simulink model "PassengerCar"  (R2019b)
settings: Solver=ode1  StartTime=0  StopTime=25  FixedStep=1.0000000000000000e-003  RelTol=1e-3
InitFcn:
  | sampleTime = str2double(get_param(bdroot, 'FixedStep'));
undefined symbols (not defined in the file or in its folder): AccPedalPos, BrakePedalPos, BrakeSwitch, DiscIntNeverNeededParam, DYNA4, EngSpd, IgnitionSwitch, InitialGear, InitialSpeed, IntendedEngTrq, LeftIndicator, MainBrakePress, MaxGear, MDL, MinGear, RefAcc, RefLane, RefLatPos, RefPath, RefPathCurv, RefSpd, RefSpdPreview, RefSpdRetrospect, RightIndicator, SteeringWheelAng, SteeringWheelTrq, UserDefinedRefValue, vm_const
libraries: UtilitiesLibrary x31, simulink x18, WheelSystemModules x13, LongitudinalControllerModules x13, LateralControllerModules x7, AnimationBusselectorModules x5, EnvironmentModules x5, BasicEngineControlModules x5, MiscellaneousControlModules x5, Animation3Modules x4, AuxiliariesModules x4, TireModules x4
(part 35 of 39)

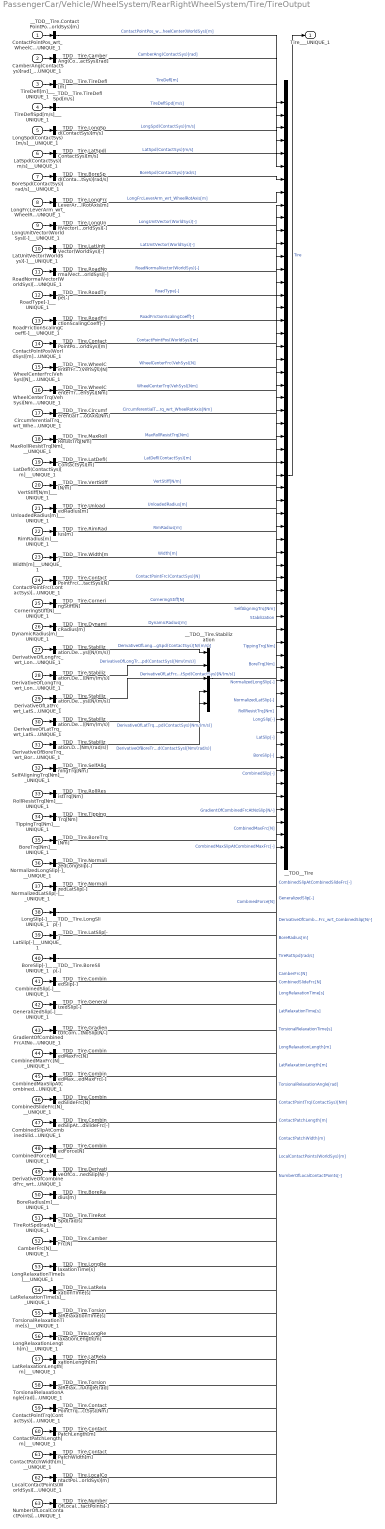
== system PassengerCar/Vehicle/WheelSystem/RearRightWheelSystem/Tire/TireOutput ==
  ContactPointPos_wrt_WheelCenter(WorldSys)[m]___UNIQUE_1 : Inport  Description=|  PortDimensions=[3]
      | <name>ContactPointPos_wrt_WheelCenter(WorldSys)[m]</name>
      | <comment></comment>
  CamberAng(ContactSys)[rad]___UNIQUE_1 : Inport  Description=|  Port=2  PortDimensions=[1]
      | <name>CamberAng(ContactSys)[rad]</name>
      | <comment></comment>
  TireDefl[m]___UNIQUE_1 : Inport  Description=|  Port=3  PortDimensions=[1]
      | <name>TireDefl[m]</name>
      | <comment></comment>
  TireDeflSpd[m/s]___UNIQUE_1 : Inport  Description=|  Port=4  PortDimensions=[1]
      | <name>TireDeflSpd[m/s]</name>
      | <comment></comment>
  LongSpd(ContactSys)[m/s]___UNIQUE_1 : Inport  Description=|  Port=5  PortDimensions=[1]
      | <name>LongSpd(ContactSys)[m/s]</name>
      | <comment></comment>
  LatSpd(ContactSys)[m/s]___UNIQUE_1 : Inport  Description=|  Port=6  PortDimensions=[1]
      | <name>LatSpd(ContactSys)[m/s]</name>
      | <comment></comment>
  BoreSpd(ContactSys)[rad/s]___UNIQUE_1 : Inport  Description=|  Port=7  PortDimensions=[1]
      | <name>BoreSpd(ContactSys)[rad/s]</name>
      | <comment></comment>
  LongFrcLeverArm_wrt_WheelRotAxis[m]___UNIQUE_1 : Inport  Description=|  Port=8  PortDimensions=[1]
      | <name>LongFrcLeverArm_wrt_WheelRotAxis[m]</name>
      | <comment></comment>
  LongUnitVector(WorldSys)[-]___UNIQUE_1 : Inport  Description=|  Port=9  PortDimensions=[3]
      | <name>LongUnitVector(WorldSys)[-]</name>
      | <comment></comment>
  LatUnitVector(WorldSys)[-]___UNIQUE_1 : Inport  Description=|  Port=10  PortDimensions=[3]
      | <name>LatUnitVector(WorldSys)[-]</name>
      | <comment></comment>
  RoadNormalVector(WorldSys)[-]___UNIQUE_1 : Inport  Description=|  Port=11  PortDimensions=[3]
      | <name>RoadNormalVector(WorldSys)[-]</name>
      | <comment></comment>
  RoadType[-]___UNIQUE_1 : Inport  Description=|  Port=12  PortDimensions=[1]
      | <name>RoadType[-]</name>
      | <comment></comment>
  RoadFrictionScalingCoeff[-]___UNIQUE_1 : Inport  Description=|  Port=13  PortDimensions=[1]
      | <name>RoadFrictionScalingCoeff[-]</name>
      | <comment></comment>
  ContactPointPos(WorldSys)[m]___UNIQUE_1 : Inport  Description=|  Port=14  PortDimensions=[3]
      | <name>ContactPointPos(WorldSys)[m]</name>
      | <comment></comment>
  WheelCenterFrc(VehSys)[N]___UNIQUE_1 : Inport  Description=|  Port=15  PortDimensions=[3]
      | <name>WheelCenterFrc(VehSys)[N]</name>
      | <comment></comment>
  WheelCenterTrq(VehSys)[Nm]___UNIQUE_1 : Inport  Description=|  Port=16  PortDimensions=[3]
      | <name>WheelCenterTrq(VehSys)[Nm]</name>
      | <comment></comment>
  CircumferentialTrq_wrt_WheelRotAxis[Nm]___UNIQUE_1 : Inport  Description=|  Port=17  PortDimensions=[1]
      | <name>CircumferentialTrq_wrt_WheelRotAxis[Nm]</name>
      | <comment></comment>
  MaxRollResistTrq[Nm]___UNIQUE_1 : Inport  Description=|  Port=18  PortDimensions=[1]
      | <name>MaxRollResistTrq[Nm]</name>
      | <comment></comment>
  LatDefl(ContactSys)[m]___UNIQUE_1 : Inport  Description=|  Port=19  PortDimensions=[1]
      | <name>LatDefl(ContactSys)[m]</name>
      | <comment></comment>
  VertStiff[N/m]___UNIQUE_1 : Inport  Description=|  Port=20  PortDimensions=[1]
      | <name>VertStiff[N/m]</name>
      | <comment></comment>
  UnloadedRadius[m]___UNIQUE_1 : Inport  Description=|  Port=21  PortDimensions=[1]
      | <name>UnloadedRadius[m]</name>
      | <comment></comment>
  RimRadius[m]___UNIQUE_1 : Inport  Description=|  Port=22  PortDimensions=[1]
      | <name>RimRadius[m]</name>
      | <comment></comment>
  Width[m]___UNIQUE_1 : Inport  Description=|  Port=23  PortDimensions=[1]
      | <name>Width[m]</name>
      | <comment></comment>
  ContactPointFrc(ContactSys)[N]___UNIQUE_1 : Inport  Description=|  Port=24  PortDimensions=[3]
      | <name>ContactPointFrc(ContactSys)[N]</name>
      | <comment></comment>
  CorneringStiff[N]___UNIQUE_1 : Inport  Description=|  Port=25  PortDimensions=[1]
      | <name>CorneringStiff[N]</name>
      | <comment></comment>
  DynamicRadius[m]___UNIQUE_1 : Inport  Description=|  Port=26  PortDimensions=[1]
      | <name>DynamicRadius[m]</name>
      | <comment></comment>
  DerivativeOfLongFrc_wrt_LongSpd(ContactSys)[N/(m/s)]___UNIQUE_1 : Inport  Description=|  Port=27  PortDimensions=[1]
      | <name>Stabilization.DerivativeOfLongFrc_wrt_LongSpd(ContactSys)[N/(m/s)]</name>
      | <comment></comment>
  DerivativeOfLongTrq_wrt_LongSpd(ContactSys)[Nm/(m/s)]___UNIQUE_1 : Inport  Description=|  Port=28  PortDimensions=[1]
      | <name>Stabilization.DerivativeOfLongTrq_wrt_LongSpd(ContactSys)[Nm/(m/s)]</name>
      | <comment></comment>
  DerivativeOfLatFrc_wrt_LatSpd(ContactSys)[N/(m/s)]___UNIQUE_1 : Inport  Description=|  Port=29  PortDimensions=[1]
      | <name>Stabilization.DerivativeOfLatFrc_wrt_LatSpd(ContactSys)[N/(m/s)]</name>
      | <comment></comment>
  DerivativeOfLatTrq_wrt_LatSpd(ContactSys)[Nm/(m/s)]___UNIQUE_1 : Inport  Description=|  Port=30  PortDimensions=[1]
      | <name>Stabilization.DerivativeOfLatTrq_wrt_LatSpd(ContactSys)[Nm/(m/s)]</name>
      | <comment></comment>
  DerivativeOfBoreTrq_wrt_BoreSpd(ContactSys)[Nm/(rad/s)]___UNIQUE_1 : Inport  Description=|  Port=31  PortDimensions=[1]
      | <name>Stabilization.DerivativeOfBoreTrq_wrt_BoreSpd(ContactSys)[Nm/(rad/s)]</name>
      | <comment></comment>
  SelfAligningTrq[Nm]___UNIQUE_1 : Inport  Description=|  Port=32  PortDimensions=[1]
      | <name>SelfAligningTrq[Nm]</name>
      | <comment></comment>
  RollResistTrq[Nm]___UNIQUE_1 : Inport  Description=|  Port=33  PortDimensions=[1]
      | <name>RollResistTrq[Nm]</name>
      | <comment></comment>
  TippingTrq[Nm]___UNIQUE_1 : Inport  Description=|  Port=34  PortDimensions=[1]
      | <name>TippingTrq[Nm]</name>
      | <comment></comment>
  BoreTrq[Nm]___UNIQUE_1 : Inport  Description=|  Port=35  PortDimensions=[1]
      | <name>BoreTrq[Nm]</name>
      | <comment></comment>
  NormalizedLongSlip[-]___UNIQUE_1 : Inport  Description=|  Port=36  PortDimensions=[1]
      | <name>NormalizedLongSlip[-]</name>
      | <comment></comment>
  NormalizedLatSlip[-]___UNIQUE_1 : Inport  Description=|  Port=37  PortDimensions=[1]
      | <name>NormalizedLatSlip[-]</name>
      | <comment></comment>
  LongSlip[-]___UNIQUE_1 : Inport  Description=|  Port=38  PortDimensions=[1]
      | <name>LongSlip[-]</name>
      | <comment></comment>
  LatSlip[-]___UNIQUE_1 : Inport  Description=|  Port=39  PortDimensions=[1]
      | <name>LatSlip[-]</name>
      | <comment></comment>
  BoreSlip[-]___UNIQUE_1 : Inport  Description=|  Port=40  PortDimensions=[1]
      | <name>BoreSlip[-]</name>
      | <comment></comment>
  CombinedSlip[-]___UNIQUE_1 : Inport  Description=|  Port=41  PortDimensions=[1]
      | <name>CombinedSlip[-]</name>
      | <comment></comment>
  GeneralizedSlip[-]___UNIQUE_1 : Inport  Description=|  Port=42  PortDimensions=[1]
      | <name>GeneralizedSlip[-]</name>
      | <comment></comment>
  GradientOfCombinedFrcAtNoSlip[N/-]___UNIQUE_1 : Inport  Description=|  Port=43  PortDimensions=[1]
      | <name>GradientOfCombinedFrcAtNoSlip[N/-]</name>
      | <comment></comment>
  CombinedMaxFrc[N]___UNIQUE_1 : Inport  Description=|  Port=44  PortDimensions=[1]
      | <name>CombinedMaxFrc[N]</name>
      | <comment></comment>
  CombinedMaxSlipAtCombinedMaxFrc[-]___UNIQUE_1 : Inport  Description=|  Port=45  PortDimensions=[1]
      | <name>CombinedMaxSlipAtCombinedMaxFrc[-]</name>
      | <comment></comment>
  CombinedSlideFrc[N]___UNIQUE_1 : Inport  Description=|  Port=46  PortDimensions=[1]
      | <name>CombinedSlideFrc[N]</name>
      | <comment></comment>
  CombinedSlipAtCombinedSlideFrc[-]___UNIQUE_1 : Inport  Description=|  Port=47  PortDimensions=[1]
      | <name>CombinedSlipAtCombinedSlideFrc[-]</name>
      | <comment></comment>
  CombinedForce[N]___UNIQUE_1 : Inport  Description=|  Port=48  PortDimensions=[1]
      | <name>CombinedForce[N]</name>
      | <comment></comment>
  DerivativeOfCombinedFrc_wrt_CombinedSlip[N/-]___UNIQUE_1 : Inport  Description=|  Port=49  PortDimensions=[1]
      | <name>DerivativeOfCombinedFrc_wrt_CombinedSlip[N/-]</name>
      | <comment></comment>
  BoreRadius[m]___UNIQUE_1 : Inport  Description=|  Port=50  PortDimensions=[1]
      | <name>BoreRadius[m]</name>
      | <comment></comment>
  TireRotSpd[rad/s]___UNIQUE_1 : Inport  Description=|  Port=51  PortDimensions=[1]
      | <name>TireRotSpd[rad/s]</name>
      | <comment></comment>
  CamberFrc[N]___UNIQUE_1 : Inport  Description=|  Port=52  PortDimensions=[1]
      | <name>CamberFrc[N]</name>
      | <comment></comment>
  LongRelaxationTime[s]___UNIQUE_1 : Inport  Description=|  Port=53  PortDimensions=[1]
      | <name>LongRelaxationTime[s]</name>
      | <comment></comment>
  LatRelaxationTime[s]___UNIQUE_1 : Inport  Description=|  Port=54  PortDimensions=[1]
      | <name>LatRelaxationTime[s]</name>
      | <comment></comment>
  TorsionalRelaxationTime[s]___UNIQUE_1 : Inport  Description=|  Port=55  PortDimensions=[1]
      | <name>TorsionalRelaxationTime[s]</name>
      | <comment></comment>
  LongRelaxationLength[m]___UNIQUE_1 : Inport  Description=|  Port=56  PortDimensions=[1]
      | <name>LongRelaxationLength[m]</name>
      | <comment></comment>
  LatRelaxationLength[m]___UNIQUE_1 : Inport  Description=|  Port=57  PortDimensions=[1]
      | <name>LatRelaxationLength[m]</name>
      | <comment></comment>
  TorsionalRelaxationAngle[rad]___UNIQUE_1 : Inport  Description=|  Port=58  PortDimensions=[1]
      | <name>TorsionalRelaxationAngle[rad]</name>
      | <comment></comment>
  ContactPointTrq(ContactSys)[Nm]___UNIQUE_1 : Inport  Description=|  Port=59  PortDimensions=[3]
      | <name>ContactPointTrq(ContactSys)[Nm]</name>
      | <comment></comment>
  ContactPatchLength[m]___UNIQUE_1 : Inport  Description=|  Port=60  PortDimensions=[1]
      | <name>ContactPatchLength[m]</name>
      | <comment></comment>
  ContactPatchWidth[m]___UNIQUE_1 : Inport  Description=|  Port=61  PortDimensions=[1]
      | <name>ContactPatchWidth[m]</name>
      | <comment></comment>
  LocalContactPoints(WorldSys)[m]___UNIQUE_1 : Inport  Description=|  Port=62  PortDimensions=[12]
      | <name>LocalContactPoints(WorldSys)[m]</name>
      | <comment></comment>
  NumberOfLocalContactPoints[-]___UNIQUE_1 : Inport  Description=|  Port=63  PortDimensions=[1]
      | <name>NumberOfLocalContactPoints[-]</name>
      | <comment></comment>
  __TDD__Tire.BoreRadius[m] : Demux  Outputs=[1]
  __TDD__Tire.BoreSlip[-] : Demux  Outputs=[1]
  __TDD__Tire.BoreSpd(ContactSys)[rad/s] : Demux  Outputs=[1]
  __TDD__Tire.BoreTrq[Nm] : Demux  Outputs=[1]
  __TDD__Tire.CamberAng(ContactSys)[rad] : Demux  Outputs=[1]
  __TDD__Tire.CamberFrc[N] : Demux  Outputs=[1]
  __TDD__Tire.CircumferentialTrq_wrt_WheelRotAxis[Nm] : Demux  Outputs=[1]
  __TDD__Tire.CombinedForce[N] : Demux  Outputs=[1]
  __TDD__Tire.CombinedMaxFrc[N] : Demux  Outputs=[1]
  __TDD__Tire.CombinedMaxSlipAtCombinedMaxFrc[-] : Demux  Outputs=[1]
  __TDD__Tire.CombinedSlideFrc[N] : Demux  Outputs=[1]
  __TDD__Tire.CombinedSlipAtCombinedSlideFrc[-] : Demux  Outputs=[1]
  __TDD__Tire.CombinedSlip[-] : Demux  Outputs=[1]
  __TDD__Tire.ContactPatchLength[m] : Demux  Outputs=[1]
  __TDD__Tire.ContactPatchWidth[m] : Demux  Outputs=[1]
  __TDD__Tire.ContactPointFrc(ContactSys)[N] : Demux  Outputs=[3]
  __TDD__Tire.ContactPointPos(WorldSys)[m] : Demux  Outputs=[3]
  __TDD__Tire.ContactPointPos_wrt_WheelCenter(WorldSys)[m] : Demux  Outputs=[3]
  __TDD__Tire.ContactPointTrq(ContactSys)[Nm] : Demux  Outputs=[3]
  __TDD__Tire.CorneringStiff[N] : Demux  Outputs=[1]
  __TDD__Tire.DerivativeOfCombinedFrc_wrt_CombinedSlip[N/-] : Demux  Outputs=[1]
  __TDD__Tire.DynamicRadius[m] : Demux  Outputs=[1]
  __TDD__Tire.GeneralizedSlip[-] : Demux  Outputs=[1]
  __TDD__Tire.GradientOfCombinedFrcAtNoSlip[N/-] : Demux  Outputs=[1]
  __TDD__Tire.LatDefl(ContactSys)[m] : Demux  Outputs=[1]
  __TDD__Tire.LatRelaxationLength[m] : Demux  Outputs=[1]
  __TDD__Tire.LatRelaxationTime[s] : Demux  Outputs=[1]
  __TDD__Tire.LatSlip[-] : Demux  Outputs=[1]
  __TDD__Tire.LatSpd(ContactSys)[m/s] : Demux  Outputs=[1]
  __TDD__Tire.LatUnitVector(WorldSys)[-] : Demux  Outputs=[3]
  __TDD__Tire.LocalContactPoints(WorldSys)[m] : Demux  Outputs=[12]
  __TDD__Tire.LongFrcLeverArm_wrt_WheelRotAxis[m] : Demux  Outputs=[1]
  __TDD__Tire.LongRelaxationLength[m] : Demux  Outputs=[1]
  __TDD__Tire.LongRelaxationTime[s] : Demux  Outputs=[1]
  __TDD__Tire.LongSlip[-] : Demux  Outputs=[1]
  __TDD__Tire.LongSpd(ContactSys)[m/s] : Demux  Outputs=[1]
  __TDD__Tire.LongUnitVector(WorldSys)[-] : Demux  Outputs=[3]
  __TDD__Tire.MaxRollResistTrq[Nm] : Demux  Outputs=[1]
  __TDD__Tire.NormalizedLatSlip[-] : Demux  Outputs=[1]
  __TDD__Tire.NormalizedLongSlip[-] : Demux  Outputs=[1]
  __TDD__Tire.NumberOfLocalContactPoints[-] : Demux  Outputs=[1]
  __TDD__Tire.RimRadius[m] : Demux  Outputs=[1]
  __TDD__Tire.RoadFrictionScalingCoeff[-] : Demux  Outputs=[1]
  __TDD__Tire.RoadNormalVector(WorldSys)[-] : Demux  Outputs=[3]
  __TDD__Tire.RoadType[-] : Demux  Outputs=[1]
  __TDD__Tire.RollResistTrq[Nm] : Demux  Outputs=[1]
  __TDD__Tire.SelfAligningTrq[Nm] : Demux  Outputs=[1]
  __TDD__Tire.Stabilization.DerivativeOfBoreTrq_wrt_BoreSpd(ContactSys)[Nm/(rad/s)] : Demux  Outputs=[1]
  __TDD__Tire.Stabilization.DerivativeOfLatFrc_wrt_LatSpd(ContactSys)[N/(m/s)] : Demux  Outputs=[1]
  __TDD__Tire.Stabilization.DerivativeOfLatTrq_wrt_LatSpd(ContactSys)[Nm/(m/s)] : Demux  Outputs=[1]
  __TDD__Tire.Stabilization.DerivativeOfLongFrc_wrt_LongSpd(ContactSys)[N/(m/s)] : Demux  Outputs=[1]
  __TDD__Tire.Stabilization.DerivativeOfLongTrq_wrt_LongSpd(ContactSys)[Nm/(m/s)] : Demux  Outputs=[1]
  __TDD__Tire.TippingTrq[Nm] : Demux  Outputs=[1]
  __TDD__Tire.TireDeflSpd[m/s] : Demux  Outputs=[1]
  __TDD__Tire.TireDefl[m] : Demux  Outputs=[1]
  __TDD__Tire.TireRotSpd[rad/s] : Demux  Outputs=[1]
  __TDD__Tire.TorsionalRelaxationAngle[rad] : Demux  Outputs=[1]
  __TDD__Tire.TorsionalRelaxationTime[s] : Demux  Outputs=[1]
  __TDD__Tire.UnloadedRadius[m] : Demux  Outputs=[1]
  __TDD__Tire.VertStiff[N/m] : Demux  Outputs=[1]
  __TDD__Tire.WheelCenterFrc(VehSys)[N] : Demux  Outputs=[3]
  __TDD__Tire.WheelCenterTrq(VehSys)[Nm] : Demux  Outputs=[3]
  __TDD__Tire.Width[m] : Demux  Outputs=[1]
  __TDO__Tire : BusCreator  Inputs=59
  __TDO__Tire.Stabilization : BusCreator  Inputs=5
  Tire___UNIQUE_1 : Outport  Description=|  PortDimensions=[92]  VectorParamsAs1DForOutWhenUnconnected=off
      | <name>ContactPointPos_wrt_WheelCenter(WorldSys)[m]</name>
      | <comment></comment>
  wires:
  ContactPointPos_wrt_WheelCenter(WorldSys)[m]___UNIQUE_1/1 -> __TDD__Tire.ContactPointPos_wrt_WheelCenter(WorldSys)[m]/1
  __TDD__Tire.ContactPointPos_wrt_WheelCenter(WorldSys)[m]/1 -> __TDO__Tire/1  "ContactPointPos_wrt_WheelCenter(WorldSys)[m]"
  CamberAng(ContactSys)[rad]___UNIQUE_1/1 -> __TDD__Tire.CamberAng(ContactSys)[rad]/1
  __TDD__Tire.CamberAng(ContactSys)[rad]/1 -> __TDO__Tire/2  "CamberAng(ContactSys)[rad]"
  TireDefl[m]___UNIQUE_1/1 -> __TDD__Tire.TireDefl[m]/1
  __TDD__Tire.TireDefl[m]/1 -> __TDO__Tire/3  "TireDefl[m]"
  TireDeflSpd[m/s]___UNIQUE_1/1 -> __TDD__Tire.TireDeflSpd[m/s]/1
  __TDD__Tire.TireDeflSpd[m/s]/1 -> __TDO__Tire/4  "TireDeflSpd[m/s]"
  LongSpd(ContactSys)[m/s]___UNIQUE_1/1 -> __TDD__Tire.LongSpd(ContactSys)[m/s]/1
  __TDD__Tire.LongSpd(ContactSys)[m/s]/1 -> __TDO__Tire/5  "LongSpd(ContactSys)[m/s]"
  LatSpd(ContactSys)[m/s]___UNIQUE_1/1 -> __TDD__Tire.LatSpd(ContactSys)[m/s]/1
  __TDD__Tire.LatSpd(ContactSys)[m/s]/1 -> __TDO__Tire/6  "LatSpd(ContactSys)[m/s]"
  BoreSpd(ContactSys)[rad/s]___UNIQUE_1/1 -> __TDD__Tire.BoreSpd(ContactSys)[rad/s]/1
  __TDD__Tire.BoreSpd(ContactSys)[rad/s]/1 -> __TDO__Tire/7  "BoreSpd(ContactSys)[rad/s]"
  LongFrcLeverArm_wrt_WheelRotAxis[m]___UNIQUE_1/1 -> __TDD__Tire.LongFrcLeverArm_wrt_WheelRotAxis[m]/1
  __TDD__Tire.LongFrcLeverArm_wrt_WheelRotAxis[m]/1 -> __TDO__Tire/8  "LongFrcLeverArm_wrt_WheelRotAxis[m]"
  LongUnitVector(WorldSys)[-]___UNIQUE_1/1 -> __TDD__Tire.LongUnitVector(WorldSys)[-]/1
  __TDD__Tire.LongUnitVector(WorldSys)[-]/1 -> __TDO__Tire/9  "LongUnitVector(WorldSys)[-]"
  LatUnitVector(WorldSys)[-]___UNIQUE_1/1 -> __TDD__Tire.LatUnitVector(WorldSys)[-]/1
  __TDD__Tire.LatUnitVector(WorldSys)[-]/1 -> __TDO__Tire/10  "LatUnitVector(WorldSys)[-]"
  RoadNormalVector(WorldSys)[-]___UNIQUE_1/1 -> __TDD__Tire.RoadNormalVector(WorldSys)[-]/1
  __TDD__Tire.RoadNormalVector(WorldSys)[-]/1 -> __TDO__Tire/11  "RoadNormalVector(WorldSys)[-]"
  RoadType[-]___UNIQUE_1/1 -> __TDD__Tire.RoadType[-]/1
  __TDD__Tire.RoadType[-]/1 -> __TDO__Tire/12  "RoadType[-]"
  RoadFrictionScalingCoeff[-]___UNIQUE_1/1 -> __TDD__Tire.RoadFrictionScalingCoeff[-]/1
  __TDD__Tire.RoadFrictionScalingCoeff[-]/1 -> __TDO__Tire/13  "RoadFrictionScalingCoeff[-]"
  ContactPointPos(WorldSys)[m]___UNIQUE_1/1 -> __TDD__Tire.ContactPointPos(WorldSys)[m]/1
  __TDD__Tire.ContactPointPos(WorldSys)[m]/1 -> __TDO__Tire/14  "ContactPointPos(WorldSys)[m]"
  WheelCenterFrc(VehSys)[N]___UNIQUE_1/1 -> __TDD__Tire.WheelCenterFrc(VehSys)[N]/1
  __TDD__Tire.WheelCenterFrc(VehSys)[N]/1 -> __TDO__Tire/15  "WheelCenterFrc(VehSys)[N]"
  WheelCenterTrq(VehSys)[Nm]___UNIQUE_1/1 -> __TDD__Tire.WheelCenterTrq(VehSys)[Nm]/1
  __TDD__Tire.WheelCenterTrq(VehSys)[Nm]/1 -> __TDO__Tire/16  "WheelCenterTrq(VehSys)[Nm]"
  CircumferentialTrq_wrt_WheelRotAxis[Nm]___UNIQUE_1/1 -> __TDD__Tire.CircumferentialTrq_wrt_WheelRotAxis[Nm]/1
  __TDD__Tire.CircumferentialTrq_wrt_WheelRotAxis[Nm]/1 -> __TDO__Tire/17  "CircumferentialTrq_wrt_WheelRotAxis[Nm]"
  MaxRollResistTrq[Nm]___UNIQUE_1/1 -> __TDD__Tire.MaxRollResistTrq[Nm]/1
  __TDD__Tire.MaxRollResistTrq[Nm]/1 -> __TDO__Tire/18  "MaxRollResistTrq[Nm]"
  LatDefl(ContactSys)[m]___UNIQUE_1/1 -> __TDD__Tire.LatDefl(ContactSys)[m]/1
  __TDD__Tire.LatDefl(ContactSys)[m]/1 -> __TDO__Tire/19  "LatDefl(ContactSys)[m]"
  VertStiff[N/m]___UNIQUE_1/1 -> __TDD__Tire.VertStiff[N/m]/1
  __TDD__Tire.VertStiff[N/m]/1 -> __TDO__Tire/20  "VertStiff[N/m]"
  UnloadedRadius[m]___UNIQUE_1/1 -> __TDD__Tire.UnloadedRadius[m]/1
  __TDD__Tire.UnloadedRadius[m]/1 -> __TDO__Tire/21  "UnloadedRadius[m]"
  RimRadius[m]___UNIQUE_1/1 -> __TDD__Tire.RimRadius[m]/1
  __TDD__Tire.RimRadius[m]/1 -> __TDO__Tire/22  "RimRadius[m]"
  Width[m]___UNIQUE_1/1 -> __TDD__Tire.Width[m]/1
  __TDD__Tire.Width[m]/1 -> __TDO__Tire/23  "Width[m]"
  ContactPointFrc(ContactSys)[N]___UNIQUE_1/1 -> __TDD__Tire.ContactPointFrc(ContactSys)[N]/1
  __TDD__Tire.ContactPointFrc(ContactSys)[N]/1 -> __TDO__Tire/24  "ContactPointFrc(ContactSys)[N]"
  CorneringStiff[N]___UNIQUE_1/1 -> __TDD__Tire.CorneringStiff[N]/1
  __TDD__Tire.CorneringStiff[N]/1 -> __TDO__Tire/25  "CorneringStiff[N]"
  DynamicRadius[m]___UNIQUE_1/1 -> __TDD__Tire.DynamicRadius[m]/1
  __TDD__Tire.DynamicRadius[m]/1 -> __TDO__Tire/26  "DynamicRadius[m]"
  DerivativeOfLongFrc_wrt_LongSpd(ContactSys)[N/(m/s)]___UNIQUE_1/1 -> __TDD__Tire.Stabilization.DerivativeOfLongFrc_wrt_LongSpd(ContactSys)[N/(m/s)]/1
  __TDD__Tire.Stabilization.DerivativeOfLongFrc_wrt_LongSpd(ContactSys)[N/(m/s)]/1 -> __TDO__Tire.Stabilization/1  "DerivativeOfLongFrc_wrt_LongSpd(ContactSys)[N/(m/s)]"
  __TDO__Tire.Stabilization/1 -> __TDO__Tire/27  "Stabilization"
  DerivativeOfLongTrq_wrt_LongSpd(ContactSys)[Nm/(m/s)]___UNIQUE_1/1 -> __TDD__Tire.Stabilization.DerivativeOfLongTrq_wrt_LongSpd(ContactSys)[Nm/(m/s)]/1
  __TDD__Tire.Stabilization.DerivativeOfLongTrq_wrt_LongSpd(ContactSys)[Nm/(m/s)]/1 -> __TDO__Tire.Stabilization/2  "DerivativeOfLongTrq_wrt_LongSpd(ContactSys)[Nm/(m/s)]"
  DerivativeOfLatFrc_wrt_LatSpd(ContactSys)[N/(m/s)]___UNIQUE_1/1 -> __TDD__Tire.Stabilization.DerivativeOfLatFrc_wrt_LatSpd(ContactSys)[N/(m/s)]/1
  __TDD__Tire.Stabilization.DerivativeOfLatFrc_wrt_LatSpd(ContactSys)[N/(m/s)]/1 -> __TDO__Tire.Stabilization/3  "DerivativeOfLatFrc_wrt_LatSpd(ContactSys)[N/(m/s)]"
  DerivativeOfLatTrq_wrt_LatSpd(ContactSys)[Nm/(m/s)]___UNIQUE_1/1 -> __TDD__Tire.Stabilization.DerivativeOfLatTrq_wrt_LatSpd(ContactSys)[Nm/(m/s)]/1
  __TDD__Tire.Stabilization.DerivativeOfLatTrq_wrt_LatSpd(ContactSys)[Nm/(m/s)]/1 -> __TDO__Tire.Stabilization/4  "DerivativeOfLatTrq_wrt_LatSpd(ContactSys)[Nm/(m/s)]"
  DerivativeOfBoreTrq_wrt_BoreSpd(ContactSys)[Nm/(rad/s)]___UNIQUE_1/1 -> __TDD__Tire.Stabilization.DerivativeOfBoreTrq_wrt_BoreSpd(ContactSys)[Nm/(rad/s)]/1
  __TDD__Tire.Stabilization.DerivativeOfBoreTrq_wrt_BoreSpd(ContactSys)[Nm/(rad/s)]/1 -> __TDO__Tire.Stabilization/5  "DerivativeOfBoreTrq_wrt_BoreSpd(ContactSys)[Nm/(rad/s)]"
  SelfAligningTrq[Nm]___UNIQUE_1/1 -> __TDD__Tire.SelfAligningTrq[Nm]/1
  __TDD__Tire.SelfAligningTrq[Nm]/1 -> __TDO__Tire/28  "SelfAligningTrq[Nm]"
  RollResistTrq[Nm]___UNIQUE_1/1 -> __TDD__Tire.RollResistTrq[Nm]/1
  __TDD__Tire.RollResistTrq[Nm]/1 -> __TDO__Tire/29  "RollResistTrq[Nm]"
  TippingTrq[Nm]___UNIQUE_1/1 -> __TDD__Tire.TippingTrq[Nm]/1
  __TDD__Tire.TippingTrq[Nm]/1 -> __TDO__Tire/30  "TippingTrq[Nm]"
  BoreTrq[Nm]___UNIQUE_1/1 -> __TDD__Tire.BoreTrq[Nm]/1
  __TDD__Tire.BoreTrq[Nm]/1 -> __TDO__Tire/31  "BoreTrq[Nm]"
  NormalizedLongSlip[-]___UNIQUE_1/1 -> __TDD__Tire.NormalizedLongSlip[-]/1
  __TDD__Tire.NormalizedLongSlip[-]/1 -> __TDO__Tire/32  "NormalizedLongSlip[-]"
  NormalizedLatSlip[-]___UNIQUE_1/1 -> __TDD__Tire.NormalizedLatSlip[-]/1
  __TDD__Tire.NormalizedLatSlip[-]/1 -> __TDO__Tire/33  "NormalizedLatSlip[-]"
  LongSlip[-]___UNIQUE_1/1 -> __TDD__Tire.LongSlip[-]/1
  __TDD__Tire.LongSlip[-]/1 -> __TDO__Tire/34  "LongSlip[-]"
  LatSlip[-]___UNIQUE_1/1 -> __TDD__Tire.LatSlip[-]/1
  __TDD__Tire.LatSlip[-]/1 -> __TDO__Tire/35  "LatSlip[-]"
  BoreSlip[-]___UNIQUE_1/1 -> __TDD__Tire.BoreSlip[-]/1
  __TDD__Tire.BoreSlip[-]/1 -> __TDO__Tire/36  "BoreSlip[-]"
  CombinedSlip[-]___UNIQUE_1/1 -> __TDD__Tire.CombinedSlip[-]/1
  __TDD__Tire.CombinedSlip[-]/1 -> __TDO__Tire/37  "CombinedSlip[-]"
  GeneralizedSlip[-]___UNIQUE_1/1 -> __TDD__Tire.GeneralizedSlip[-]/1
  __TDD__Tire.GeneralizedSlip[-]/1 -> __TDO__Tire/38  "GeneralizedSlip[-]"
  GradientOfCombinedFrcAtNoSlip[N/-]___UNIQUE_1/1 -> __TDD__Tire.GradientOfCombinedFrcAtNoSlip[N/-]/1
  __TDD__Tire.GradientOfCombinedFrcAtNoSlip[N/-]/1 -> __TDO__Tire/39  "GradientOfCombinedFrcAtNoSlip[N/-]"
  CombinedMaxFrc[N]___UNIQUE_1/1 -> __TDD__Tire.CombinedMaxFrc[N]/1
  __TDD__Tire.CombinedMaxFrc[N]/1 -> __TDO__Tire/40  "CombinedMaxFrc[N]"
  CombinedMaxSlipAtCombinedMaxFrc[-]___UNIQUE_1/1 -> __TDD__Tire.CombinedMaxSlipAtCombinedMaxFrc[-]/1
  __TDD__Tire.CombinedMaxSlipAtCombinedMaxFrc[-]/1 -> __TDO__Tire/41  "CombinedMaxSlipAtCombinedMaxFrc[-]"
  CombinedSlideFrc[N]___UNIQUE_1/1 -> __TDD__Tire.CombinedSlideFrc[N]/1
  __TDD__Tire.CombinedSlideFrc[N]/1 -> __TDO__Tire/42  "CombinedSlideFrc[N]"
  CombinedSlipAtCombinedSlideFrc[-]___UNIQUE_1/1 -> __TDD__Tire.CombinedSlipAtCombinedSlideFrc[-]/1
  __TDD__Tire.CombinedSlipAtCombinedSlideFrc[-]/1 -> __TDO__Tire/43  "CombinedSlipAtCombinedSlideFrc[-]"
  CombinedForce[N]___UNIQUE_1/1 -> __TDD__Tire.CombinedForce[N]/1
  __TDD__Tire.CombinedForce[N]/1 -> __TDO__Tire/44  "CombinedForce[N]"
  DerivativeOfCombinedFrc_wrt_CombinedSlip[N/-]___UNIQUE_1/1 -> __TDD__Tire.DerivativeOfCombinedFrc_wrt_CombinedSlip[N/-]/1
  __TDD__Tire.DerivativeOfCombinedFrc_wrt_CombinedSlip[N/-]/1 -> __TDO__Tire/45  "DerivativeOfCombinedFrc_wrt_CombinedSlip[N/-]"
  BoreRadius[m]___UNIQUE_1/1 -> __TDD__Tire.BoreRadius[m]/1
  __TDD__Tire.BoreRadius[m]/1 -> __TDO__Tire/46  "BoreRadius[m]"
  TireRotSpd[rad/s]___UNIQUE_1/1 -> __TDD__Tire.TireRotSpd[rad/s]/1
  __TDD__Tire.TireRotSpd[rad/s]/1 -> __TDO__Tire/47  "TireRotSpd[rad/s]"
  CamberFrc[N]___UNIQUE_1/1 -> __TDD__Tire.CamberFrc[N]/1
  __TDD__Tire.CamberFrc[N]/1 -> __TDO__Tire/48  "CamberFrc[N]"
  LongRelaxationTime[s]___UNIQUE_1/1 -> __TDD__Tire.LongRelaxationTime[s]/1
  __TDD__Tire.LongRelaxationTime[s]/1 -> __TDO__Tire/49  "LongRelaxationTime[s]"
  LatRelaxationTime[s]___UNIQUE_1/1 -> __TDD__Tire.LatRelaxationTime[s]/1
  __TDD__Tire.LatRelaxationTime[s]/1 -> __TDO__Tire/50  "LatRelaxationTime[s]"
  TorsionalRelaxationTime[s]___UNIQUE_1/1 -> __TDD__Tire.TorsionalRelaxationTime[s]/1
  __TDD__Tire.TorsionalRelaxationTime[s]/1 -> __TDO__Tire/51  "TorsionalRelaxationTime[s]"
  LongRelaxationLength[m]___UNIQUE_1/1 -> __TDD__Tire.LongRelaxationLength[m]/1
  __TDD__Tire.LongRelaxationLength[m]/1 -> __TDO__Tire/52  "LongRelaxationLength[m]"
  LatRelaxationLength[m]___UNIQUE_1/1 -> __TDD__Tire.LatRelaxationLength[m]/1
  __TDD__Tire.LatRelaxationLength[m]/1 -> __TDO__Tire/53  "LatRelaxationLength[m]"
  TorsionalRelaxationAngle[rad]___UNIQUE_1/1 -> __TDD__Tire.TorsionalRelaxationAngle[rad]/1
  __TDD__Tire.TorsionalRelaxationAngle[rad]/1 -> __TDO__Tire/54  "TorsionalRelaxationAngle[rad]"
  ContactPointTrq(ContactSys)[Nm]___UNIQUE_1/1 -> __TDD__Tire.ContactPointTrq(ContactSys)[Nm]/1
  __TDD__Tire.ContactPointTrq(ContactSys)[Nm]/1 -> __TDO__Tire/55  "ContactPointTrq(ContactSys)[Nm]"
  ContactPatchLength[m]___UNIQUE_1/1 -> __TDD__Tire.ContactPatchLength[m]/1
  __TDD__Tire.ContactPatchLength[m]/1 -> __TDO__Tire/56  "ContactPatchLength[m]"
  ContactPatchWidth[m]___UNIQUE_1/1 -> __TDD__Tire.ContactPatchWidth[m]/1
  __TDD__Tire.ContactPatchWidth[m]/1 -> __TDO__Tire/57  "ContactPatchWidth[m]"
  LocalContactPoints(WorldSys)[m]___UNIQUE_1/1 -> __TDD__Tire.LocalContactPoints(WorldSys)[m]/1
  __TDD__Tire.LocalContactPoints(WorldSys)[m]/1 -> __TDO__Tire/58  "LocalContactPoints(WorldSys)[m]"
  NumberOfLocalContactPoints[-]___UNIQUE_1/1 -> __TDD__Tire.NumberOfLocalContactPoints[-]/1
  __TDD__Tire.NumberOfLocalContactPoints[-]/1 -> __TDO__Tire/59  "NumberOfLocalContactPoints[-]"
  __TDO__Tire/1 -> Tire___UNIQUE_1/1  "Tire"

== system PassengerCar/VehicleControl/LateralControl/Disabled LateralControl/ControlSystems/Control Systems Parameters ==
  CurvatureControl : Subsystem
      settings: CopyFcn=DYNA4.Internal.ModelCallbacks.Modules.UpdateMaskParameters(gcb);  NameChangeFcn=DYNA4.Internal.ModelCallbacks.Modules.UpdateMaskParameters(gcb);
  PathControl : Subsystem
      settings: CopyFcn=DYNA4.Internal.ModelCallbacks.Modules.UpdateMaskParameters(gcb);  NameChangeFcn=DYNA4.Internal.ModelCallbacks.Modules.UpdateMaskParameters(gcb);

== system PassengerCar/VehicleControl/LateralControl/Disabled LateralControl/ControlSystems/DynaSystemInfo ==

== system PassengerCar/VehicleControl/LateralControl/Disabled LateralControl/ControlSystems/Lateral Controller ==
  User-Defined Control : Subsystem  TreatAsAtomicUnit=on

== system PassengerCar/VehicleControl/LateralControl/Disabled LateralControl/ControlSystems/LateralControlOutput ==
  __SRC__LateralControl.LateralPhase : Constant  Value=0.0  OutDataTypeStr=Inherit: Inherit via back propagation
  __SRC__LateralControl.LeftIndicator : Constant  Value=0.0  OutDataTypeStr=Inherit: Inherit via back propagation
  __SRC__LateralControl.RightIndicator : Constant  Value=0.0  OutDataTypeStr=Inherit: Inherit via back propagation
  __SRC__LateralControl.SteeringWheelAng : Constant  Value=0.0  OutDataTypeStr=Inherit: Inherit via back propagation
  __SRC__LateralControl.SteeringWheelInputSwitch : Constant  Value=0.0  OutDataTypeStr=Inherit: Inherit via back propagation
  __SRC__LateralControl.SteeringWheelTrq : Constant  Value=0.0  OutDataTypeStr=Inherit: Inherit via back propagation
  __SRC__LateralControl.UserDefined1 : Constant  Value=0.0  OutDataTypeStr=Inherit: Inherit via back propagation
  __SRC__LateralControl.UserDefined2 : Constant  Value=0.0  OutDataTypeStr=Inherit: Inherit via back propagation
  __SRC__LateralControl.UserDefinedRefValue : Constant  Value=0.0  OutDataTypeStr=Inherit: Inherit via back propagation
  __TDO__LateralControl : BusCreator  Inputs=9
  LateralControl___UNIQUE_1 : Outport  Description=|  PortDimensions=[9]  VectorParamsAs1DForOutWhenUnconnected=off
      | <name>SteeringWheelAng</name>
      | <comment>Steering wheel angle</comment>
  wires:
  __TDO__LateralControl/1 -> LateralControl___UNIQUE_1/1  "LateralControl"
  __SRC__LateralControl.UserDefined2/1 -> __TDO__LateralControl/9  "UserDefined2[-]"
  __SRC__LateralControl.UserDefined1/1 -> __TDO__LateralControl/8  "UserDefined1[-]"
  __SRC__LateralControl.LateralPhase/1 -> __TDO__LateralControl/7  "LateralPhase[-]"
  __SRC__LateralControl.RightIndicator/1 -> __TDO__LateralControl/6  "RightIndicator[0;1]"
  __SRC__LateralControl.LeftIndicator/1 -> __TDO__LateralControl/5  "LeftIndicator[0;1]"
  __SRC__LateralControl.UserDefinedRefValue/1 -> __TDO__LateralControl/4  "UserDefinedRefValue[-]"
  __SRC__LateralControl.SteeringWheelInputSwitch/1 -> __TDO__LateralControl/3  "SteeringWheelInputSwitch[-]"
  __SRC__LateralControl.SteeringWheelTrq/1 -> __TDO__LateralControl/2  "SteeringWheelTrq[Nm]"
  __SRC__LateralControl.SteeringWheelAng/1 -> __TDO__LateralControl/1  "SteeringWheelAng[rad]"

== system PassengerCar/VehicleControl/LateralControl/Disabled LateralControl/ControlSystemsPreprocessor/Maneuver ==
  DynaModuleInfo : Subsystem  Tag=DynaModuleInfo
      mask init:
      | data = get_param(gcb, 'UserData');
      mask Display: disp(['Type = ', data.type, '\nName = ', char(data.name)]);

== system PassengerCar/VehicleControl/LateralControl/Enabled LateralControl/ControlSystems/Control Systems Parameters ==
  note: TASK_LAT_STEERING_WHEEL_ANG = 1;
      | 	TASK_LAT_STEERING_WHEEL_TORQUE = 2;
      | 	TASK_LAT_PATH_CONTROL = 3;
      | 	TASK_LAT_CURVATURE_CONTROL = 4;
      | 	TASK_LAT_USER_DEFINED = 5;
  TaskIdentifier : Inport
  CtrlSystemsAbscissae : Inport  Port=2
  Bus Selector : BusSelector  OutputSignals=Task
  CurvatureControl : LateralControllerModules/DataContainerCurvatureControl  DATA_NODE=MDL.VehicleControl.LateralControl.ControlSystems.CurvatureControl  PreviewDist=MDL.VehicleControl.LateralControl.ControlSystems.CurvatureControl.PreviewDist  PreviewTime=MDL.VehicleControl.LateralControl.ControlSystems.CurvatureControl.PreviewTime  TargetAimDist=MDL.VehicleControl.LateralControl.ControlSystems.CurvatureControl.TargetAimDist  MaxLeftSteeringRate=MDL.VehicleControl.LateralControl.ControlSystems.CurvatureControl.MaxLeftSteeringRate  MaxRightSteeringRate=MDL.VehicleControl.LateralControl.ControlSystems.CurvatureControl.MaxRightSteeringRate  SteeringAngSmoothTimeConst=MDL.VehicleControl.LateralControl.ControlSystems.CurvatureControl.SteeringAngSmoothTimeConst  LatCtrlGain=MDL.VehicleControl.LateralControl.ControlSystems.CurvatureControl.LatCtrlGain  ControllerDeviationScaling=MDL.VehicleControl.LateralControl.ControlSystems.CurvatureControl.ControllerDeviationScaling  FrontAxleLatStiff=MDL.VehicleControl.LateralControl.ControlSystems.CurvatureControl.FrontAxleLatStiff  RearAxleLatStiff=MDL.VehicleControl.LateralControl.ControlSystems.CurvatureControl.RearAxleLatStiff  RearTiresLatFrcSmoothTimeConst=MDL.VehicleControl.LateralControl.ControlSystems.CurvatureControl.RearTiresLatFrcSmoothTimeConst  RearTiresLatFrcSwitch=MDL.VehicleControl.LateralControl.ControlSystems.CurvatureControl.RearTiresLatFrcSwitch  RearTiresLatFrcScaling=MDL.VehicleControl.LateralControl.ControlSystems.CurvatureControl.RearTiresLatFrcScaling  SmoothingInterval=MDL.VehicleControl.LateralControl.ControlSystems.CurvatureControl.SmoothingInterval  Preview=MDL.VehicleControl.LateralControl.ControlSystems.CurvatureControl.Preview  DrivingSkill=MDL.VehicleControl.LateralControl.ControlSystems.CurvatureControl.DrivingSkill  Smoothness=MDL.VehicleControl.LateralControl.ControlSystems.CurvatureControl.Smoothness
  Merge : Merge
  PathControl : LateralControllerModules/DataContainerPathControl  DATA_NODE=MDL.VehicleControl.LateralControl.ControlSystems.PathControl  PreviewDist=MDL.VehicleControl.LateralControl.ControlSystems.PathControl.PreviewDist  PreviewTime=MDL.VehicleControl.LateralControl.ControlSystems.PathControl.PreviewTime  TargetAimDist=MDL.VehicleControl.LateralControl.ControlSystems.PathControl.TargetAimDist  MaxLeftSteeringRate=MDL.VehicleControl.LateralControl.ControlSystems.PathControl.MaxLeftSteeringRate  MaxRightSteeringRate=MDL.VehicleControl.LateralControl.ControlSystems.PathControl.MaxRightSteeringRate  SteeringAngSmoothTimeConst=MDL.VehicleControl.LateralControl.ControlSystems.PathControl.SteeringAngSmoothTimeConst  LatCtrlGain=MDL.VehicleControl.LateralControl.ControlSystems.PathControl.LatCtrlGain  ControllerDeviationScaling=MDL.VehicleControl.LateralControl.ControlSystems.PathControl.ControllerDeviationScaling  FrontAxleLatStiff=MDL.VehicleControl.LateralControl.ControlSystems.PathControl.FrontAxleLatStiff  RearAxleLatStiff=MDL.VehicleControl.LateralControl.ControlSystems.PathControl.RearAxleLatStiff  RearTiresLatFrcSmoothTimeConst=MDL.VehicleControl.LateralControl.ControlSystems.PathControl.RearTiresLatFrcSmoothTimeConst  RearTiresLatFrcSwitch=MDL.VehicleControl.LateralControl.ControlSystems.PathControl.RearTiresLatFrcSwitch  RearTiresLatFrcScaling=MDL.VehicleControl.LateralControl.ControlSystems.PathControl.RearTiresLatFrcScaling  LaneChangeDurationTime=MDL.VehicleControl.LateralControl.ControlSystems.PathControl.LaneChangeDurationTime  LaneChangeDurationDist=MDL.VehicleControl.LateralControl.ControlSystems.PathControl.LaneChangeDurationDist  SmoothingInterval=MDL.VehicleControl.LateralControl.ControlSystems.PathControl.SmoothingInterval  Preview=MDL.VehicleControl.LateralControl.ControlSystems.PathControl.Preview  DrivingSkill=MDL.VehicleControl.LateralControl.ControlSystems.PathControl.DrivingSkill  Smoothness=MDL.VehicleControl.LateralControl.ControlSystems.PathControl.Smoothness
  Switch Case : SwitchCase  CaseConditions={vm_const('TASK_LAT_PATH_CONTROL'), vm_const('TASK_LAT_CURVATURE_CONTROL')}  ShowDefaultCase=off
  ControllerParameters : Outport  VectorParamsAs1DForOutWhenUnconnected=off
  wires:
  Switch Case/2 -> CurvatureControl/Action
  Switch Case/1 -> PathControl/Action
  CtrlSystemsAbscissae/1 -> CurvatureControl/1, PathControl/1
  Merge/1 -> ControllerParameters/1
  CurvatureControl/1 -> Merge/2
  PathControl/1 -> Merge/1
  TaskIdentifier/1 -> Bus Selector/1
  Bus Selector/1 -> Switch Case/1  "<Task>"

== system PassengerCar/VehicleControl/LateralControl/Enabled LateralControl/ControlSystems/DynaSystemInfo ==

== system PassengerCar/VehicleControl/LateralControl/Enabled LateralControl/ControlSystems/Lateral Controller ==
  note: TASK_LAT_STEERING_WHEEL_ANG = 1;
      | 	TASK_LAT_STEERING_WHEEL_TORQUE = 2;
      | 	TASK_LAT_PATH_CONTROL = 3;
      | 	TASK_LAT_CURVATURE_CONTROL = 4;
      | 	TASK_LAT_USER_DEFINED = 5;
  TaskIdentifiers : Inport
  SourceIdentifiers : Inport  Port=2
  ControlInputs : Inport  Port=3
  ControllerParameters : Inport  Port=4
  VehicleInfo : Inport  Port=5
  Bus Selector : BusSelector  OutputSignals=Task,Subtask
  Initialization : Subsystem
  Merge : Merge  Inputs=5
  Path and Curvature Control : Subsystem  TreatAsAtomicUnit=on
  Steering Wheel Angle Input : Subsystem  TreatAsAtomicUnit=on
  Steering Wheel Torque Input : Subsystem  TreatAsAtomicUnit=on
  Switch Case : SwitchCase  CaseConditions={vm_const('TASK_LAT_STEERING_WHEEL_ANG'), vm_const('TASK_LAT_STEERING_WHEEL_TORQUE'), [vm_const('TASK_LAT_PATH_CONTROL'),vm_const('TASK_LAT_CURVATURE_CONTROL')], vm_const('TASK_LAT_USER_DEFINED')}
  User-Defined Control : Subsystem  TreatAsAtomicUnit=on
  SteeringWheelDemands : Outport  VectorParamsAs1DForOutWhenUnconnected=off
  UserDefinedRefValue[-] : Outport  Port=2  PortDimensions=1  VectorParamsAs1DForOutWhenUnconnected=off
  wires:
  Steering Wheel Torque Input/1(SteeringWheelDemands) -> Merge/2
  Switch Case/2 -> Steering Wheel Torque Input/Action
  User-Defined Control/1(SteeringWheelDemands) -> Merge/4
  Path and Curvature Control/1(SteeringWheelDemands) -> Merge/3
  Initialization/1(SteeringWheelDemands) -> Merge/5
  Switch Case/3 -> Path and Curvature Control/Action
  Switch Case/4 -> User-Defined Control/Action
  Switch Case/1 -> Steering Wheel Angle Input/Action
  Switch Case/5 -> Initialization/Action
  User-Defined Control/2(UserDefinedRefValue[-]) -> UserDefinedRefValue[-]/1
  SourceIdentifiers/1 -> User-Defined Control/3(SourceIdentifiers)
  ControlInputs/1 -> Steering Wheel Angle Input/1(ControlInputs), Steering Wheel Torque Input/1(ControlInputs), Path and Curvature Control/1(ControlInputs), User-Defined Control/1(ControlInputs)
  ControllerParameters/1 -> Path and Curvature Control/2(ControllerParameters)
  VehicleInfo/1 -> Path and Curvature Control/3(VehicleInfo), User-Defined Control/2(VehicleInfo), Steering Wheel Angle Input/2(VehicleInfo), Steering Wheel Torque Input/2(VehicleInfo)
  Merge/1 -> SteeringWheelDemands/1
  Steering Wheel Angle Input/1(SteeringWheelDemands) -> Merge/1
  TaskIdentifiers/1 -> Bus Selector/1
  Bus Selector/1 -> Switch Case/1  "<Task>"
  Bus Selector/2 -> User-Defined Control/4(SubtaskIdentifiers)  "<Subtask>"

== system PassengerCar/VehicleControl/LateralControl/Enabled LateralControl/ControlSystems/LateralControlOutput ==
  SteeringWheelAng[rad]___UNIQUE_1 : Inport  Description=|  PortDimensions=[1]
      | <name>SteeringWheelAng[rad]</name>
      | <comment>Steering wheel angle</comment>
  SteeringWheelTrq[Nm]___UNIQUE_1 : Inport  Description=|  Port=2  PortDimensions=[1]
      | <name>SteeringWheelTrq[Nm]</name>
      | <comment>Steering wheel torque</comment>
  SteeringWheelInputSwitch[-]___UNIQUE_1 : Inport  Description=|  Port=3  PortDimensions=[1]
      | <name>SteeringWheelInputSwitch[-]</name>
      | <comment>Steering wheel input switch (0: angle, 1: torque)</comment>
  UserDefinedRefValue[-]___UNIQUE_1 : Inport  Description=|  Port=4  PortDimensions=[1]
      | <name>UserDefinedRefValue[-]</name>
      | <comment>User-defined reference value</comment>
  LeftIndicator[0;1]___UNIQUE_1 : Inport  Description=|  Port=5  PortDimensions=[1]
      | <name>LeftIndicator[0;1]</name>
      | <comment>Left indicator state</comment>
  RightIndicator[0;1]___UNIQUE_1 : Inport  Description=|  Port=6  PortDimensions=[1]
      | <name>RightIndicator[0;1]</name>
      | <comment>Right indicator state</comment>
  LateralPhase[-]___UNIQUE_1 : Inport  Description=|  Port=7  PortDimensions=[1]
      | <name>LateralPhase[-]</name>
      | <comment>Lateral phase number</comment>
  UserDefined1[-]___UNIQUE_1 : Inport  Description=|  Port=8  PortDimensions=[1]
      | <name>UserDefined.UserDefined1[-]</name>
      | <comment>User-defined additional input 1 (can be edited by the user)</comment>
  UserDefined2[-]___UNIQUE_1 : Inport  Description=|  Port=9  PortDimensions=[1]
      | <name>UserDefined.UserDefined2[-]</name>
      | <comment>User-defined additional input 2 (can be edited by the user)</comment>
  __TDD__LateralControl.LateralPhase[-] : Demux  Outputs=[1]
  __TDD__LateralControl.LeftIndicator[0;1] : Demux  Outputs=[1]
  __TDD__LateralControl.RightIndicator[0;1] : Demux  Outputs=[1]
  __TDD__LateralControl.SteeringWheelAng[rad] : Demux  Outputs=[1]
  __TDD__LateralControl.SteeringWheelInputSwitch[-] : Demux  Outputs=[1]
  __TDD__LateralControl.SteeringWheelTrq[Nm] : Demux  Outputs=[1]
  __TDD__LateralControl.UserDefined1[-] : Demux  Outputs=[1]
  __TDD__LateralControl.UserDefined2[-] : Demux  Outputs=[1]
  __TDD__LateralControl.UserDefinedRefValue[-] : Demux  Outputs=[1]
  __TDO__LateralControl : BusCreator  Inputs=9
  LateralControl___UNIQUE_1 : Outport  Description=|  PortDimensions=[9]  VectorParamsAs1DForOutWhenUnconnected=off
      | <name>SteeringWheelAng[rad]</name>
      | <comment>Steering wheel angle</comment>
  wires:
  __TDO__LateralControl/1 -> LateralControl___UNIQUE_1/1  "LateralControl"
  __TDD__LateralControl.UserDefined2[-]/1 -> __TDO__LateralControl/9  "UserDefined2[-]"
  UserDefined2[-]___UNIQUE_1/1 -> __TDD__LateralControl.UserDefined2[-]/1  "UserDefined2[-]"
  __TDD__LateralControl.UserDefined1[-]/1 -> __TDO__LateralControl/8  "UserDefined1[-]"
  UserDefined1[-]___UNIQUE_1/1 -> __TDD__LateralControl.UserDefined1[-]/1  "UserDefined1[-]"
  __TDD__LateralControl.LateralPhase[-]/1 -> __TDO__LateralControl/7  "LateralPhase[-]"
  LateralPhase[-]___UNIQUE_1/1 -> __TDD__LateralControl.LateralPhase[-]/1  "LateralPhase[-]"
  __TDD__LateralControl.RightIndicator[0;1]/1 -> __TDO__LateralControl/6  "RightIndicator[0;1]"
  RightIndicator[0;1]___UNIQUE_1/1 -> __TDD__LateralControl.RightIndicator[0;1]/1  "RightIndicator[0;1]"
  __TDD__LateralControl.LeftIndicator[0;1]/1 -> __TDO__LateralControl/5  "LeftIndicator[0;1]"
  LeftIndicator[0;1]___UNIQUE_1/1 -> __TDD__LateralControl.LeftIndicator[0;1]/1  "LeftIndicator[0;1]"
  __TDD__LateralControl.UserDefinedRefValue[-]/1 -> __TDO__LateralControl/4  "UserDefinedRefValue[-]"
  UserDefinedRefValue[-]___UNIQUE_1/1 -> __TDD__LateralControl.UserDefinedRefValue[-]/1  "UserDefinedRefValue[-]"
  __TDD__LateralControl.SteeringWheelInputSwitch[-]/1 -> __TDO__LateralControl/3  "SteeringWheelInputSwitch[-]"
  SteeringWheelInputSwitch[-]___UNIQUE_1/1 -> __TDD__LateralControl.SteeringWheelInputSwitch[-]/1  "SteeringWheelInputSwitch[-]"
  __TDD__LateralControl.SteeringWheelTrq[Nm]/1 -> __TDO__LateralControl/2  "SteeringWheelTrq[Nm]"
  SteeringWheelTrq[Nm]___UNIQUE_1/1 -> __TDD__LateralControl.SteeringWheelTrq[Nm]/1  "SteeringWheelTrq[Nm]"
  __TDD__LateralControl.SteeringWheelAng[rad]/1 -> __TDO__LateralControl/1  "SteeringWheelAng[rad]"
  SteeringWheelAng[rad]___UNIQUE_1/1 -> __TDD__LateralControl.SteeringWheelAng[rad]/1  "SteeringWheelAng[rad]"

== system PassengerCar/VehicleControl/LateralControl/Enabled LateralControl/ControlSystems/SteeringWheelLimitation ==
  SteeringWheelDemands : Inport
  ControlInputs : Inport  Port=2
  Bus Selector1 : BusSelector  OutputSignals=MaxSteeringWheelRateLeft,MaxSteeringWheelRateRight,MaxSteeringWheelAngLeft,MaxSteeringWheelAngRight
  Bus Selector2 : BusSelector  OutputSignals=SteeringWheelAng[rad]
  LimitSteeringWheelAng : simulink/Discontinuities/Saturation Dynamic  OutMin=[]  OutMax=[]  OutDataTypeStr=Inherit: Same as second input  OutDataType=fixdt(1, 16)  OutScaling=2^-10  DoSatur=off
  LimitSteeringWheelGradient : simulink/Discontinuities/Rate Limiter Dynamic
      settings: SourceProductName=Simulink
  ModifiedSteeringWhlAng[rad] : Outport  VectorParamsAs1DForOutWhenUnconnected=off
  wires:
  Bus Selector2/1 -> LimitSteeringWheelGradient/2  "<SteeringWheelAng[rad]>"
  Bus Selector1/4 -> LimitSteeringWheelAng/3  "<MaxSteeringWheelAngRight>"
  Bus Selector1/3 -> LimitSteeringWheelAng/1  "<MaxSteeringWheelAngLeft>"
  Bus Selector1/2 -> LimitSteeringWheelGradient/3  "<MaxSteeringWheelRateRight>"
  Bus Selector1/1 -> LimitSteeringWheelGradient/1  "<MaxSteeringWheelRateLeft>"
  SteeringWheelDemands/1 -> Bus Selector2/1
  LimitSteeringWheelGradient/1 -> LimitSteeringWheelAng/2
  ControlInputs/1 -> Bus Selector1/1
  LimitSteeringWheelAng/1 -> ModifiedSteeringWhlAng[rad]/1  "SteeringWheelAng[rad]"

== system PassengerCar/VehicleControl/LateralControl/Enabled LateralControl/ControlSystemsPreprocessor/External Presetting of Controller  ==
  TaskIdentifiers : Inport
  SourceIdentifiers : Inport  Port=2
  ExtCtrlVariablesEnforced : Inport  Port=3
  Presetting Source Identifiers : Subsystem
  Presetting Task Identifiers : Subsystem
  ModifiedTaskIdentifiers : Outport  VectorParamsAs1DForOutWhenUnconnected=off
  ModifiedSourceIdentifiers : Outport  Port=2  VectorParamsAs1DForOutWhenUnconnected=off
  wires:
  Presetting Source Identifiers/1(ModifiedSourceIdentifiers) -> ModifiedSourceIdentifiers/1
  ExtCtrlVariablesEnforced/1 -> Presetting Task Identifiers/2("ExternalControlVariablesEnforced "), Presetting Source Identifiers/1("ExternalControlVariablesEnforced ")
  TaskIdentifiers/1 -> Presetting Task Identifiers/1(TaskIdentifiers)
  Presetting Task Identifiers/1(ModifiedTaskIdentifiers) -> ModifiedTaskIdentifiers/1
  SourceIdentifiers/1 -> Presetting Source Identifiers/2(SourceIdentifiers)

== system PassengerCar/VehicleControl/LateralControl/Enabled LateralControl/ControlSystemsPreprocessor/Generation of Guidance Data ==
  note: TASK_LAT_STEERING_WHEEL_ANG = 1;
      | 	TASK_LAT_STEERING_WHEEL_TORQUE = 2;
      | 	TASK_LAT_PATH_CONTROL = 3;
      | 	TASK_LAT_CURVATURE_CONTROL = 4;
      | 	TASK_LAT_USER_DEFINED = 5;
  TaskIdentifiers : Inport
  ControlInputs : Inport  Port=2
  ControllerParameters : Inport  Port=3
  VehicleInfo : Inport  Port=4
  Bus Creator : BusCreator  Inputs=20
  Bus Selector2 : BusSelector  OutputSignals=SteeringWheelAng,SteeringWheelTrq,RefLatPos,RefLane,RefPath,RefPathCurv,UserDefinedRefValue,LeftIndicator,RightIndicator,MaxSteeringWheelAngLeft,MaxSteeringWheelAngRight,MaxSteeringWheelRateLeft,MaxSteeringWheelRateRight
  Bus Selector6 : BusSelector  OutputSignals=Subtask,Task
  CurvatureGuidance : LateralControllerModules/CurvatureGuidance  sample_time=-1
  Demux : Demux  Outputs=7
  "Initialization, SteeringWheel, UserDefined" : Subsystem
  Merge : Merge  Inputs=3
  Mux : Mux  Inputs=2
  PathGuidance : LateralControllerModules/PathGuidance  sample_time=-1
  PreviousSubtask : Memory  InheritSampleTime=on
  Switch Case : SwitchCase  CaseConditions={vm_const('TASK_LAT_PATH_CONTROL'),vm_const('TASK_LAT_CURVATURE_CONTROL')}
  ExtendedControlInputs : Outport  VectorParamsAs1DForOutWhenUnconnected=off
  wires:
  [IRoadInterface] -> CurvatureGuidance/1, PathGuidance/1
  Bus Selector2/13 -> Bus Creator/20  "<MaxSteeringWheelRateRight>"
  Bus Selector2/12 -> Bus Creator/19  "<MaxSteeringWheelRateLeft>"
  Bus Selector2/2 -> Bus Creator/9  "<SteeringWheelTrq>"
  Bus Selector2/3 -> Bus Creator/10  "<RefLatPos>"
  Bus Selector2/11 -> Bus Creator/18  "<MaxSteeringWheelAngRight>"
  Bus Selector2/10 -> Bus Creator/17  "<MaxSteeringWheelAngLeft>"
  Bus Selector2/4 -> Bus Creator/11  "<RefLane>"
  Bus Selector2/9 -> Bus Creator/16  "<RightIndicator>"
  Bus Selector2/5 -> Bus Creator/12  "<RefPath>"
  Bus Selector2/8 -> Bus Creator/15  "<LeftIndicator>"
  Bus Selector2/6 -> Bus Creator/13  "<RefPathCurv>"
  Bus Selector2/7 -> Bus Creator/14  "<UserDefinedRefValue>"
  "Initialization, SteeringWheel, UserDefined"/1(TargetAndTargetAim) -> Merge/3
  PreviousSubtask/1 -> Mux/2
  Mux/1 -> PathGuidance/2, CurvatureGuidance/2
  Merge/1 -> Demux/1
  CurvatureGuidance/1 -> Merge/2
  PathGuidance/1 -> Merge/1
  Bus Creator/1 -> ExtendedControlInputs/1
  Switch Case/3 -> "Initialization, SteeringWheel, UserDefined"/Action
  Switch Case/2 -> CurvatureGuidance/Action
  Switch Case/1 -> PathGuidance/Action
  Bus Selector6/1 -> PreviousSubtask/1, Mux/1  "<Subtask>"
  Bus Selector6/2 -> Switch Case/1  "<Task>"
  TaskIdentifiers/1 -> Bus Selector6/1
  ControllerParameters/1 -> CurvatureGuidance/4, PathGuidance/4
  VehicleInfo/1 -> PathGuidance/5, CurvatureGuidance/5
  ControlInputs/1 -> CurvatureGuidance/3, Bus Selector2/1, PathGuidance/3
  Bus Selector2/1 -> Bus Creator/8  "<SteeringWheelAng>"
  Demux/1 -> Bus Creator/1  "tgt_x"
  Demux/2 -> Bus Creator/2  "tgt_y"
  Demux/3 -> Bus Creator/3  "tgt_z"
  Demux/4 -> Bus Creator/4  "tgt_cu"
  Demux/5 -> Bus Creator/5  "tgt_psi"
  Demux/6 -> Bus Creator/6  "taim_x"
  Demux/7 -> Bus Creator/7  "taim_y"

== system PassengerCar/VehicleControl/LateralControl/Enabled LateralControl/ControlSystemsPreprocessor/Generation of Hold Data ==
  PhaseTrigger : Inport
  LatCTRL : Inport  Port=2
  VehicleInfo : Inport  Port=3
  Bus Selector18 : BusSelector  OutputSignals=VehicleRoadInfo_RoadQ[m],VehicleRoadInfo_LaneID[-],VehicleRoadInfo_LaneCurvature[1/m]  OutputAsBus=on
  Enabled Subsystem : Subsystem  TreatAsAtomicUnit=on
  Memory : Memory  InheritSampleTime=on
  Memory1 : Memory  InheritSampleTime=on
  HoldData : Outport  VectorParamsAs1DForOutWhenUnconnected=off
  wires:
  Memory1/1 -> Enabled Subsystem/2(VehicleInfo)
  Memory/1 -> Enabled Subsystem/1(LatCTRL)
  Bus Selector18/1 -> Memory1/1
  VehicleInfo/1 -> Bus Selector18/1
  Enabled Subsystem/1(HoldData) -> HoldData/1
  LatCTRL/1 -> Memory/1
  PhaseTrigger/1 -> Enabled Subsystem/Enable
